simulink model "storage_tank_validated2019b"  (R2019b)
settings: Solver=VariableStepAuto  StartTime=0.0  StopTime=10.0  RelTol=1e-3
values from neighbouring files (symbols this model uses):
  A_tank = 3/12    (= 0.25)    [storage_tank_constants.m]
  Acoil = 3.6/4    (= 0.9)    [storage_tank_constants.m]
  delt = 10^5    (= 100000)    [storage_tank_constants.m]
  U_loss = 0.5    [storage_tank_constants.m]
  Ucoil = 250    [storage_tank_constants.m]
  vol_coil = 0.014/4    (= 0.0035)    [storage_tank_constants.m]
settings Model: Creator=Mariana  LastModifiedBy=Mariana

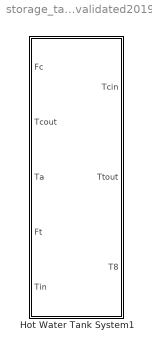
== system storage_tank_validated2019b ==
  Hot Water Tank System1 : Subsystem
      mask Display: image('hot_water_tank.PNG');

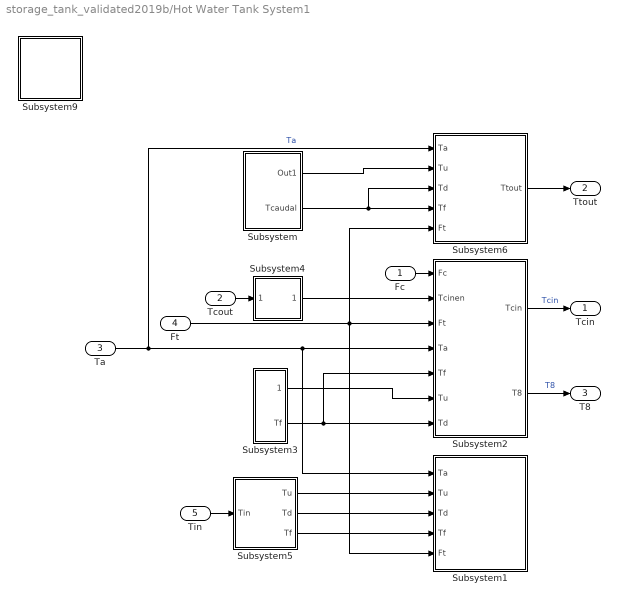
== system storage_tank_validated2019b/Hot Water Tank System1 ==
  "Fc " : Inport
  "Tcout " : Inport  Port=2
  Ta : Inport  Port=3
  Ft : Inport  Port=4
  "Tin " : Inport  Port=5
  Subsystem : Subsystem
  Subsystem1 : Subsystem
  Subsystem2 : Subsystem
  Subsystem3 : Subsystem
  Subsystem4 : Subsystem
  Subsystem5 : Subsystem
  Subsystem6 : Subsystem
  Subsystem9 : Subsystem
  "Tcin " : Outport
  Ttout : Outport  Port=2
  T8 : Outport  Port=3
  wires:
  Subsystem2/1(Tcin) -> "Tcin "/1  "Tcin"
  "Fc "/1 -> Subsystem2/1("Fc ")
  Subsystem/1(Out1) -> Subsystem6/2(Tu)
  Subsystem/2("Tcaudal ") -> Subsystem6/3(Td), Subsystem6/4("Tf ")
  "Tin "/1 -> Subsystem5/1(Tin)
  Subsystem3/1(Out2) -> Subsystem2/6(Tu)
  Subsystem3/2("Tf ") -> Subsystem2/5("Tf "), Subsystem2/7(Td)
  Subsystem4/1(Out1) -> Subsystem2/2("Tcinen ")
  Subsystem5/1(Tu) -> Subsystem1/2(Tu)
  Subsystem5/2(Td) -> Subsystem1/3(Td)
  "Tcout "/1 -> Subsystem4/1("Tcout ")
  Ta/1 -> Subsystem1/1(Ta), Subsystem2/4(Ta), Subsystem6/1(Ta)  "Ta"
  Ft/1 -> Subsystem1/5(Ft), Subsystem6/5(Ft), Subsystem2/3(Ft)
  Subsystem5/3("Tf ") -> Subsystem1/4("Tf ")
  Subsystem6/1(Ttout) -> Ttout/1
  Subsystem2/2(T8) -> T8/1  "T8"

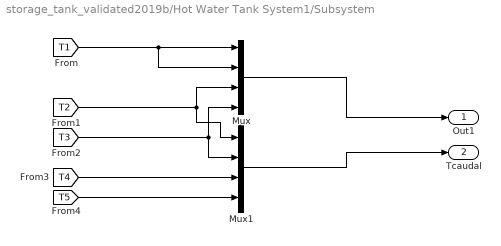
== system storage_tank_validated2019b/Hot Water Tank System1/Subsystem ==
  Mux : Mux
  Mux1 : Mux
  Out1 : Outport
  "Tcaudal " : Outport  Port=2
  wires:
  Mux1/1 -> "Tcaudal "/1
  [T1] -> Mux/2, Mux/1
  [T2] -> Mux1/1, Mux/3
  Mux/1 -> Out1/1
  [T3] -> Mux1/2, Mux/4
  [T4] -> Mux1/3
  [T5] -> Mux1/4

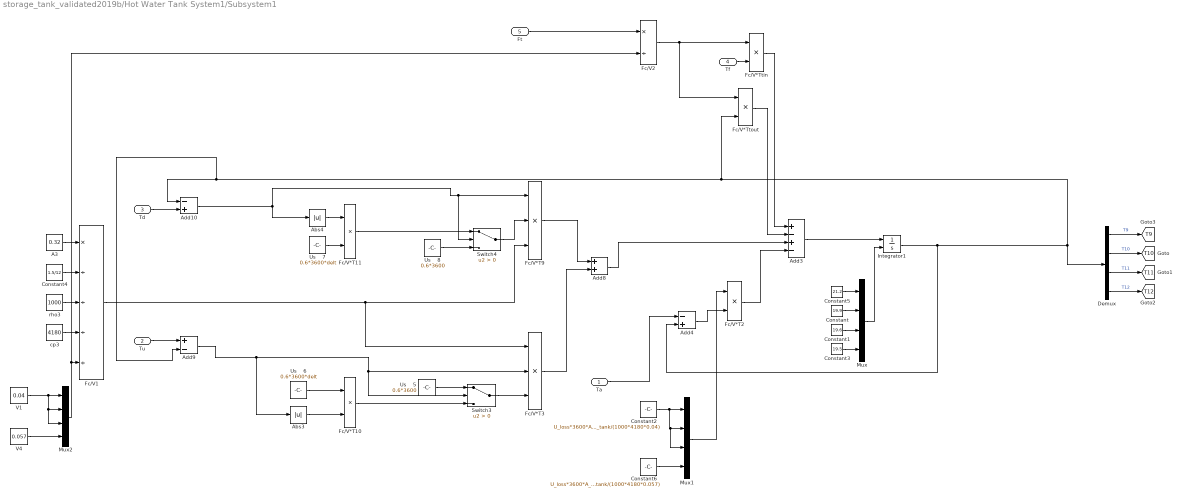
== system storage_tank_validated2019b/Hot Water Tank System1/Subsystem1 ==
  Ta : Inport
  Tu : Inport  Port=2
  Td : Inport  Port=3
  "Tf " : Inport  Port=4
  Ft : Inport  Port=5
  A3 : Constant  Value=0.32
  Abs3 : Abs  ZeroCross=off
  Abs4 : Abs  ZeroCross=off
  Add10 : Sum  Inputs=-+
  Add3 : Sum  Inputs=+-+-
  Add4 : Sum  Inputs=-+
  Add8 : Sum
  Add9 : Sum  Inputs=+-
  Constant : Constant  Value=19.9
  Constant1 : Constant  Value=19.6
  Constant2 : Constant  Value=U_loss*3600*A_tank/(1000*4180*0.04)
  Constant3 : Constant  Value=19.5
  Constant4 : Constant  Value=1.5/12
  Constant5 : Constant  Value=21.2
  Constant6 : Constant  Value=U_loss*3600*A_tank/(1000*4180*0.057)
  Demux : Demux
  Fc/V*T10 : Product  Inputs=**
  Fc/V*T11 : Product  Inputs=**
  Fc/V*T2 : Product  Inputs=**
  Fc/V*T3 : Product  Inputs=***
  Fc/V*T9 : Product  Inputs=***
  Fc/V*Ttin : Product  Inputs=**
  Fc/V*Ttout : Product  Inputs=**
  Fc/V1 : Product  Inputs=*////
  Fc/V2 : Product  Inputs=*/
  Integrator1 : Integrator  InitialConditionSource=external  InitialCondition=55.1
  Mux : Mux
  Mux1 : Mux
  Mux2 : Mux
  Switch3 : Switch  Criteria=u2 > Threshold  ZeroCross=off
  Switch4 : Switch  Criteria=u2 > Threshold  ZeroCross=off
  Us    5 : Constant  Value=0.6*3600
  Us    6 : Constant  Value=0.6*3600*delt
  Us    7 : Constant  Value=0.6*3600*delt
  Us    8 : Constant  Value=0.6*3600
  V1 : Constant  Value=0.04
  V4 : Constant  Value=0.057
  cp3 : Constant  Value=4180
  rho3 : Constant  Value=1000
  tag scope: T10=global, T11=global, T12=global, T9=global
  wires:
  Constant5/1 -> Mux/1
  Integrator1/1 -> Add4/2, Demux/1, Fc/V*Ttout/2, Add9/2, Add10/1
  Constant/1 -> Mux/2
  Demux/1 -> [T9]  "T9"
  Switch3/1 -> Fc/V*T3/3
  Add8/1 -> Add3/3
  Constant1/1 -> Mux/3
  Mux2/1 -> Fc/V2/2, Fc/V1/5
  Demux/4 -> [T12]  "T12"
  Us    6/1 -> Fc/V*T10/1
  Fc/V2/1 -> Fc/V*Ttin/1, Fc/V*Ttout/1
  rho3/1 -> Fc/V1/3
  Fc/V*Ttin/1 -> Add3/1
  Fc/V*Ttout/1 -> Add3/2
  Constant3/1 -> Mux/4
  A3/1 -> Fc/V1/1
  Abs3/1 -> Fc/V*T10/2
  Ta/1 -> Add4/1
  Switch4/1 -> Fc/V*T9/2
  Fc/V*T2/1 -> Add3/4
  Fc/V*T3/1 -> Add8/2
  Add3/1 -> Integrator1/1
  Abs4/1 -> Fc/V*T11/1
  cp3/1 -> Fc/V1/4
  Us    7/1 -> Fc/V*T11/2
  Ft/1 -> Fc/V2/1
  Fc/V*T11/1 -> Switch4/1
  Add9/1 -> Fc/V*T3/2, Switch3/2, Abs3/1
  Us    8/1 -> Switch4/3
  Fc/V*T10/1 -> Switch3/3
  Mux/1 -> Integrator1/2
  Constant4/1 -> Fc/V1/2
  Demux/2 -> [T10]  "T10"
  Add10/1 -> Switch4/2, Fc/V*T9/1, Abs4/1
  Tu/1 -> Add9/1
  Demux/3 -> [T11]  "T11"
  Td/1 -> Add10/2
  Add4/1 -> Fc/V*T2/2
  Fc/V1/1 -> Fc/V*T9/3, Fc/V*T3/1
  Us    5/1 -> Switch3/1
  "Tf "/1 -> Fc/V*Ttin/2
  Fc/V*T9/1 -> Add8/1
  V1/1 -> Mux2/3, Mux2/2, Mux2/1
  V4/1 -> Mux2/4
  Mux1/1 -> Fc/V*T2/1
  Constant2/1 -> Mux1/3, Mux1/2, Mux1/1
  Constant6/1 -> Mux1/4

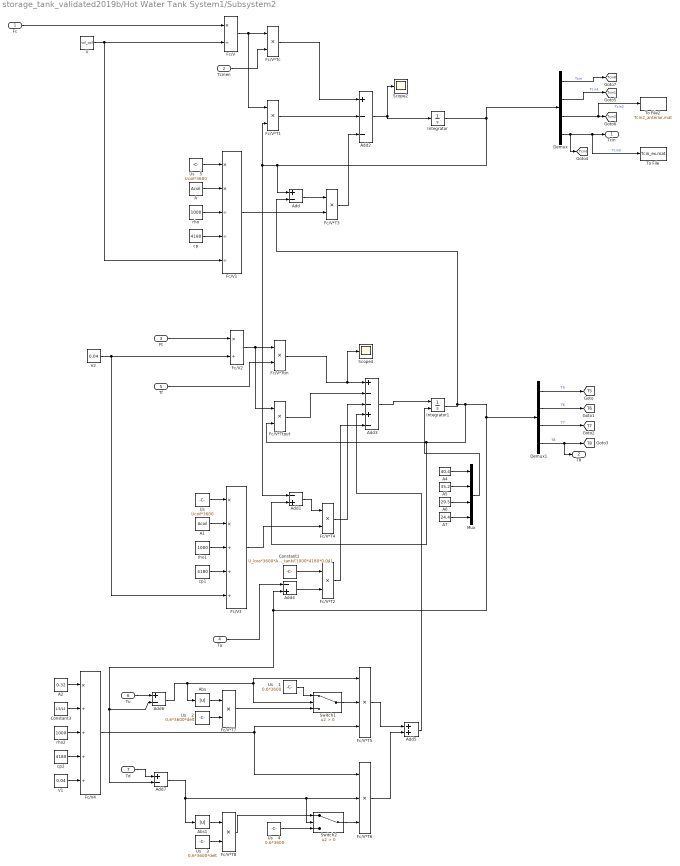
== system storage_tank_validated2019b/Hot Water Tank System1/Subsystem2 ==
  "Fc " : Inport
  "Tcinen " : Inport  Port=2
  Ft : Inport  Port=3
  Ta : Inport  Port=4
  "Tf " : Inport  Port=5
  Tu : Inport  Port=6
  Td : Inport  Port=7
  A : Constant  Value=Acoil
  A1 : Constant  Value=Acoil
  A2 : Constant  Value=0.32
  A4 : Constant  Value=40.4
  A5 : Constant  Value=35.2
  A6 : Constant  Value=29.5
  A7 : Constant  Value=24.4
  Abs : Abs  ZeroCross=off
  Abs1 : Abs  ZeroCross=off
  Add : Sum  Inputs=+-
  Add1 : Sum  Inputs=-+
  Add2 : Sum  Inputs=+--
  Add3 : Sum  Inputs=+--+-
  Add4 : Sum  Inputs=-+
  Add5 : Sum
  Add6 : Sum  Inputs=+-
  Add7 : Sum  Inputs=+-
  Constant2 : Constant  Value=U_loss*3600*A_tank/(1000*4180*0.04)
  Constant3 : Constant  Value=1.5/12
  Demux : Demux
  Demux1 : Demux
  Fc/V : Product  Inputs=*/
  Fc/V*T{1..4,7..8} (6 alike) : Product  Inputs=**
  Fc/V*T5 : Product  Inputs=***
  Fc/V*T6 : Product  Inputs=***
  Fc/V*Tc : Product  Inputs=**
  Fc/V*Ttin : Product  Inputs=**
  Fc/V*Ttout : Product  Inputs=**
  Fc/V1 : Product  Inputs=**///
  Fc/V2 : Product  Inputs=*/
  Fc/V3 : Product  Inputs=**///
  Fc/V4 : Product  Inputs=*////
  Integrator : Integrator  InitialCondition=25.7
  Integrator1 : Integrator  InitialConditionSource=external  InitialCondition=42.7
  Mux : Mux
  Scope2 : Scope
  Scope4 : Scope
  Switch1 : Switch  Criteria=u2 > Threshold  ZeroCross=off
  Switch2 : Switch  Criteria=u2 > Threshold  ZeroCross=off
  To File : ToFile  Filename=Tcin_ex.mat  MatrixName=Tcin_ex  SampleTime=1
  To File2 : ToFile  Filename=Tcin2_anterior.mat  MatrixName=Tcin2_anterior  SampleTime=1
  "Us    " : Constant  Value=Ucoil*3600
  Us    1 : Constant  Value=0.6*3600
  Us    2 : Constant  Value=0.6*3600*delt
  Us    3 : Constant  Value=0.6*3600*delt
  Us    4 : Constant  Value=0.6*3600
  Us    5 : Constant  Value=Ucoil*3600
  V : Constant  Value=vol_coil
  V1 : Constant  Value=0.04
  V2 : Constant  Value=0.04
  cp : Constant  Value=4180
  cp1 : Constant  Value=4180
  cp2 : Constant  Value=4180
  rho : Constant  Value=1000
  rho1 : Constant  Value=1000
  rho2 : Constant  Value=1000
  Tcin : Outport
  T8 : Outport  Port=2
  tag scope: T5=global, T6=global, T7=global, T8=global, Tcin0=global, Tcin1=global, Tcin2=global, Tcin3=global
  wires:
  Fc/V*T3/1 -> Add2/3
  Fc/V2/1 -> Fc/V*Ttin/1, Fc/V*Ttout/1
  Fc/V*Ttin/1 -> Scope4/1, Add3/1
  Add1/1 -> Fc/V*T4/1
  rho/1 -> Fc/V1/3
  Integrator1/1 -> Add1/2, Fc/V*Ttout/2, Add6/2, Add7/2, Add4/2, Demux1/1, Add/2
  Fc/V/1 -> Fc/V*T1/1, Fc/V*Tc/1
  Integrator/1 -> Demux/1, Add/1, Fc/V*T1/2, Add1/1
  V/1 -> Fc/V1/5, Fc/V/2
  Add2/1 -> Scope2/1, Integrator/1
  Fc/V*T1/1 -> Add2/2
  Fc/V3/1 -> Fc/V*T4/2
  Ft/1 -> Fc/V2/1
  cp/1 -> Fc/V1/4
  A1/1 -> Fc/V3/2
  Fc/V*Ttout/1 -> Add3/2
  Fc/V*T4/1 -> Add3/3
  Fc/V1/1 -> Fc/V*T3/2
  Add/1 -> Fc/V*T3/1
  Ta/1 -> Add4/1
  "Tcinen "/1 -> Fc/V*Tc/2
  rho1/1 -> Fc/V3/3
  Fc/V*Tc/1 -> Add2/1
  V2/1 -> Fc/V2/2, Fc/V3/5
  "Fc "/1 -> Fc/V/1
  Add3/1 -> Integrator1/1
  cp1/1 -> Fc/V3/4
  A/1 -> Fc/V1/2
  Add5/1 -> Add3/4
  V1/1 -> Fc/V4/5
  Fc/V4/1 -> Fc/V*T5/3, Fc/V*T6/1
  rho2/1 -> Fc/V4/3
  cp2/1 -> Fc/V4/4
  A2/1 -> Fc/V4/1
  Fc/V*T5/1 -> Add5/1
  Fc/V*T6/1 -> Add5/2
  Add7/1 -> Switch2/2, Fc/V*T6/2, Abs1/1
  Add6/1 -> Switch1/2, Fc/V*T5/1, Abs/1
  "Tf "/1 -> Fc/V*Ttin/2
  Constant3/1 -> Fc/V4/2
  Switch1/1 -> Fc/V*T5/2
  Us    1/1 -> Switch1/1
  Fc/V*T7/1 -> Switch1/3
  Switch2/1 -> Fc/V*T6/3
  Fc/V*T8/1 -> Switch2/1
  Us    4/1 -> Switch2/3
  Us    2/1 -> Fc/V*T7/2
  Us    3/1 -> Fc/V*T8/2
  Abs/1 -> Fc/V*T7/1
  Abs1/1 -> Fc/V*T8/1
  Tu/1 -> Add6/1
  Demux/1 -> [Tcin0]  "Tcin"
  Demux/2 -> [Tcin1]  "Tcin1"
  Demux/3 -> To File2/1, [Tcin2]  "Tcin2"
  Demux/4 -> [Tcin3], To File/1, Tcin/1  "Tcin3"
  Demux1/1 -> [T5]  "T5"
  Demux1/3 -> [T7]  "T7"
  Demux1/4 -> [T8], T8/1  "T8"
  Mux/1 -> Integrator1/2
  A4/1 -> Mux/1
  A5/1 -> Mux/2
  A6/1 -> Mux/3
  A7/1 -> Mux/4
  Td/1 -> Add7/1
  Demux1/2 -> [T6]  "T6"
  "Us    "/1 -> Fc/V3/1
  Us    5/1 -> Fc/V1/1
  Add4/1 -> Fc/V*T2/2
  Constant2/1 -> Fc/V*T2/1
  Fc/V*T2/1 -> Add3/5

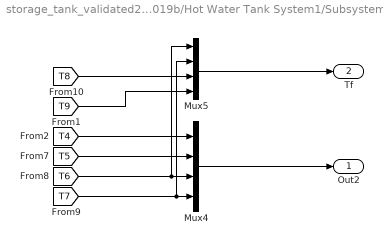
== system storage_tank_validated2019b/Hot Water Tank System1/Subsystem3 ==
  Mux4 : Mux
  Mux5 : Mux
  Out2 : Outport
  "Tf " : Outport  Port=2
  wires:
  [T6] -> Mux5/1, Mux4/3
  [T8] -> Mux5/3
  [T7] -> Mux5/2, Mux4/4
  [T5] -> Mux4/2
  Mux4/1 -> Out2/1
  [T4] -> Mux4/1
  Mux5/1 -> "Tf "/1
  [T9] -> Mux5/4

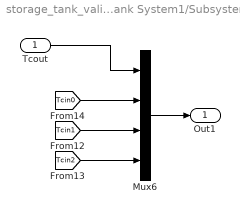
== system storage_tank_validated2019b/Hot Water Tank System1/Subsystem4 ==
  "Tcout " : Inport
  Mux6 : Mux
  Out1 : Outport
  wires:
  Mux6/1 -> Out1/1
  "Tcout "/1 -> Mux6/1
  [Tcin0] -> Mux6/2
  [Tcin1] -> Mux6/3
  [Tcin2] -> Mux6/4

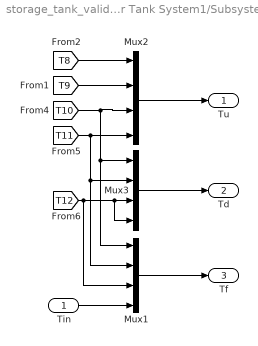
== system storage_tank_validated2019b/Hot Water Tank System1/Subsystem5 ==
  Tin : Inport
  Mux1 : Mux
  Mux2 : Mux
  Mux3 : Mux
  Tu : Outport
  Td : Outport  Port=2
  "Tf " : Outport  Port=3
  wires:
  Mux3/1 -> Td/1
  [T12] -> Mux3/3, Mux3/4, Mux1/3
  [T10] -> Mux2/3, Mux3/1, Mux1/1
  Mux2/1 -> Tu/1
  [T9] -> Mux2/2
  [T11] -> Mux2/4, Mux3/2, Mux1/2
  Mux1/1 -> "Tf "/1
  Tin/1 -> Mux1/4
  [T8] -> Mux2/1

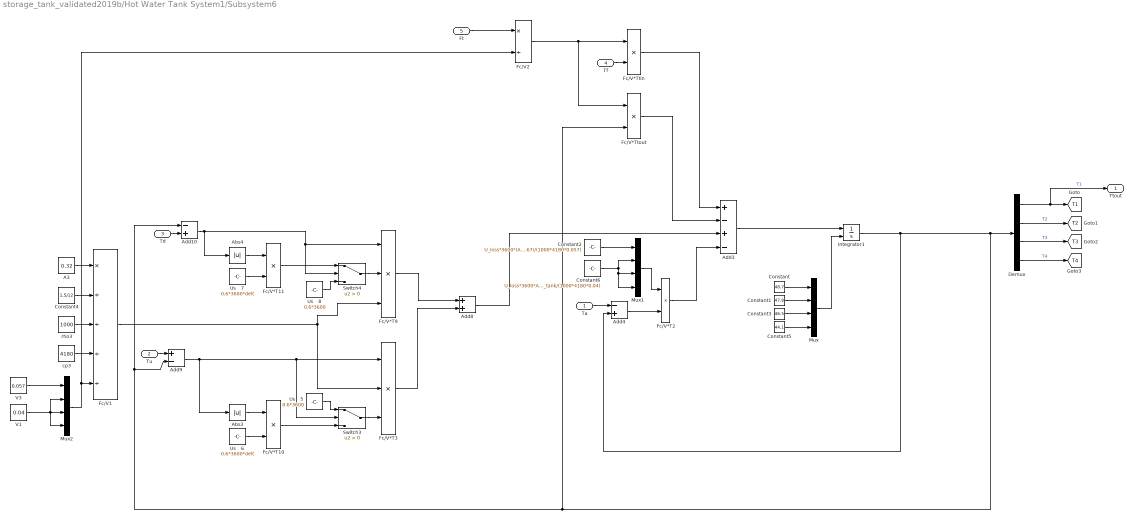
== system storage_tank_validated2019b/Hot Water Tank System1/Subsystem6 ==
  Ta : Inport
  Tu : Inport  Port=2
  Td : Inport  Port=3
  "Tf " : Inport  Port=4
  Ft : Inport  Port=5
  A3 : Constant  Value=0.32
  Abs3 : Abs  ZeroCross=off
  Abs4 : Abs  ZeroCross=off
  Add10 : Sum  Inputs=-+
  Add3 : Sum  Inputs=+-+-
  Add4 : Sum  Inputs=-+
  Add8 : Sum
  Add9 : Sum  Inputs=+-
  Constant : Constant  Value=48.7
  Constant1 : Constant  Value=47.8
  Constant2 : Constant  Value=U_loss*3600*(A_tank+0.67)/(1000*4180*0.057)
  Constant3 : Constant  Value=46.5
  Constant4 : Constant  Value=1.5/12
  Constant5 : Constant  Value=44.1
  Constant6 : Constant  Value=U_loss*3600*A_tank/(1000*4180*0.04)
  Demux : Demux
  Fc/V*T10 : Product  Inputs=**
  Fc/V*T11 : Product  Inputs=**
  Fc/V*T2 : Product  Inputs=**
  Fc/V*T3 : Product  Inputs=***
  Fc/V*T9 : Product  Inputs=***
  Fc/V*Ttin : Product  Inputs=**
  Fc/V*Ttout : Product  Inputs=**
  Fc/V1 : Product  Inputs=*////
  Fc/V2 : Product  Inputs=*/
  Integrator1 : Integrator  InitialConditionSource=external  InitialCondition=55.1
  Mux : Mux
  Mux1 : Mux
  Mux2 : Mux
  Switch3 : Switch  Criteria=u2 > Threshold  ZeroCross=off
  Switch4 : Switch  Criteria=u2 > Threshold  ZeroCross=off
  Us    5 : Constant  Value=0.6*3600
  Us    6 : Constant  Value=0.6*3600*delt
  Us    7 : Constant  Value=0.6*3600*delt
  Us    8 : Constant  Value=0.6*3600
  V1 : Constant  Value=0.04
  V3 : Constant  Value=0.057
  cp3 : Constant  Value=4180
  rho3 : Constant  Value=1000
  Ttout : Outport
  tag scope: T1=global, T2=global, T3=global, T4=global
  wires:
  Ta/1 -> Add4/1
  Add4/1 -> Fc/V*T2/2
  Add3/1 -> Integrator1/1
  Switch4/1 -> Fc/V*T9/2
  Us    5/1 -> Switch3/1
  Fc/V*T10/1 -> Switch3/3
  Add9/1 -> Fc/V*T3/1, Switch3/2, Abs3/1
  Us    6/1 -> Fc/V*T10/2
  Fc/V*T3/1 -> Add8/2
  Constant4/1 -> Fc/V1/2
  Fc/V*T11/1 -> Switch4/1
  Us    8/1 -> Switch4/3
  Us    7/1 -> Fc/V*T11/2
  A3/1 -> Fc/V1/1
  Abs3/1 -> Fc/V*T10/1
  Abs4/1 -> Fc/V*T11/1
  Fc/V*T9/1 -> Add8/1
  rho3/1 -> Fc/V1/3
  Tu/1 -> Add9/1
  Fc/V1/1 -> Fc/V*T9/3, Fc/V*T3/2
  Switch3/1 -> Fc/V*T3/3
  cp3/1 -> Fc/V1/4
  Integrator1/1 -> Add4/2, Fc/V*Ttout/2, Add10/1, Add9/2, Demux/1
  Td/1 -> Add10/2
  Add10/1 -> Abs4/1, Switch4/2, Fc/V*T9/1
  Demux/1 -> [T1], Ttout/1  "T1"
  Demux/2 -> [T2]  "T2"
  Demux/3 -> [T3]  "T3"
  Demux/4 -> [T4]  "T4"
  Mux/1 -> Integrator1/2
  Constant/1 -> Mux/1
  Constant1/1 -> Mux/2
  Constant3/1 -> Mux/3
  Constant5/1 -> Mux/4
  Ft/1 -> Fc/V2/1
  Fc/V2/1 -> Fc/V*Ttout/1, Fc/V*Ttin/1
  Mux2/1 -> Fc/V2/2, Fc/V1/5
  "Tf "/1 -> Fc/V*Ttin/2
  Add8/1 -> Add3/3
  Fc/V*Ttin/1 -> Add3/1
  Fc/V*Ttout/1 -> Add3/2
  Fc/V*T2/1 -> Add3/4
  Mux1/1 -> Fc/V*T2/1
  Constant2/1 -> Mux1/1
  Constant6/1 -> Mux1/4, Mux1/3, Mux1/2
  V3/1 -> Mux2/1
  V1/1 -> Mux2/4, Mux2/2, Mux2/3

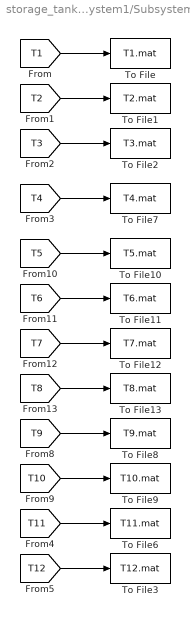
== system storage_tank_validated2019b/Hot Water Tank System1/Subsystem9 ==
  To File : ToFile  Filename=T1.mat  MatrixName=T1  SampleTime=1
  To File1 : ToFile  Filename=T2.mat  MatrixName=T2  SampleTime=1
  To File10 : ToFile  Filename=T5.mat  MatrixName=T5  SampleTime=1
  To File11 : ToFile  Filename=T6.mat  MatrixName=T6  SampleTime=1
  To File12 : ToFile  Filename=T7.mat  MatrixName=T7  SampleTime=1
  To File13 : ToFile  Filename=T8.mat  MatrixName=T8  SampleTime=1
  To File2 : ToFile  Filename=T3.mat  MatrixName=T3  SampleTime=1
  To File3 : ToFile  Filename=T12.mat  MatrixName=T12  SampleTime=1
  To File6 : ToFile  Filename=T11.mat  MatrixName=T11  SampleTime=1
  To File7 : ToFile  Filename=T4.mat  MatrixName=T4  SampleTime=1
  To File8 : ToFile  Filename=T9.mat  MatrixName=T9  SampleTime=1
  To File9 : ToFile  Filename=T10.mat  MatrixName=T10  SampleTime=1
  wires:
  [T1] -> To File/1
  [T2] -> To File1/1
  [T3] -> To File2/1
  [T9] -> To File8/1
  [T10] -> To File9/1
  [T5] -> To File10/1
  [T6] -> To File11/1
  [T7] -> To File12/1
  [T8] -> To File13/1
  [T11] -> To File6/1
  [T4] -> To File7/1
  [T12] -> To File3/1
